simulink model "Simple_Joystick_CGN"  (R2025b)
settings: Solver=FixedStepDiscrete  StartTime=0.0  StopTime=inf  RelTol=1e-3
undefined symbols (not defined in the file): pwm_zero_set
libraries: ros2lib x2
settings Model: Creator=vulcangrip  LastModifiedBy=vulcangrip
settings OptimizationCC: DefaultParameterBehavior=Inlined  EnhancedBackFolding=on  PassReuseOutputArgsAs=Individual arguments  ZeroExternalMemoryAtStartup=off  ZeroInternalMemoryAtStartup=off  MaxStackSize=64  OptimizeBlockOrder=speed  DifferentSizesBufferReuse=on  OptimizationCustomize=off  EfficientTunableParamExpr=on
settings DebuggingCC: ParameterTunabilityLossMsg=error
settings HardwareCC: ProdBitPerLong=64.0  ProdHWDeviceType=Intel->x86-64 (Linux 64)
settings SFSimCC: MATLABDynamicMemAlloc=off  SimTargetLang=C++  SimDLTargetLibrary=mkl-dnn
settings RTWCC: SystemTargetFile=ert.tlc  HardwareBoard=Robot Operating System 2 (ROS 2)  TLCOptions="-aInlineSetEventsForThisBaseRateFcn=TLC_FALSE -aSuppressMultiTaskScheduler=TLC_FALSE  -aRateBasedStepFcn=0"  GenCodeOnly=on  TemplateMakefile=ert_default_tmf  Toolchain=Colcon Tools  BuildConfiguration=Faster Runs  TargetLang=C++  CheckMdlBeforeBuild=Warning  Description=Embedded Coder
settings CodeAppCC: ForceParamTrailComments=on  IgnoreCustomStorageClasses=off  OperatorAnnotations=on  SimulinkDataObjDesc=on  SFDataObjDesc=on  InsertBlockDesc=on
settings ERTTargetCC: ExtModeTransport=2.0  ExtModeStaticAlloc=on  ExtModeAutomaticAllocSize=off  ExtModeMexFile=ext_xcp  ExtModeIntrfLevel=Level2 - Open  RootIOFormat=Structure reference  TargetLangStandard=C++11 (ISO)  CodeInterfacePackaging=C++ class  SubcomponentCodeInterfacePackaging=C++ class

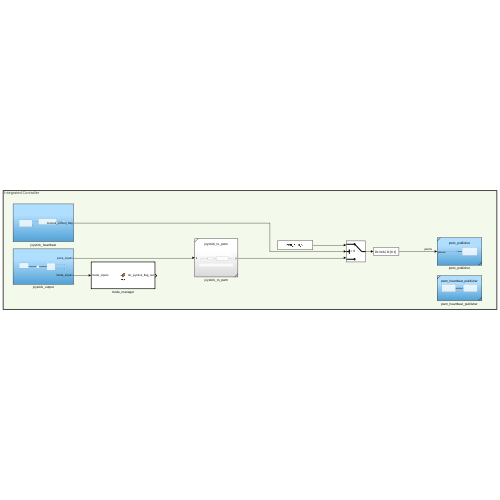
[thumbnail: Simulink's stored preview of the top-level diagram]
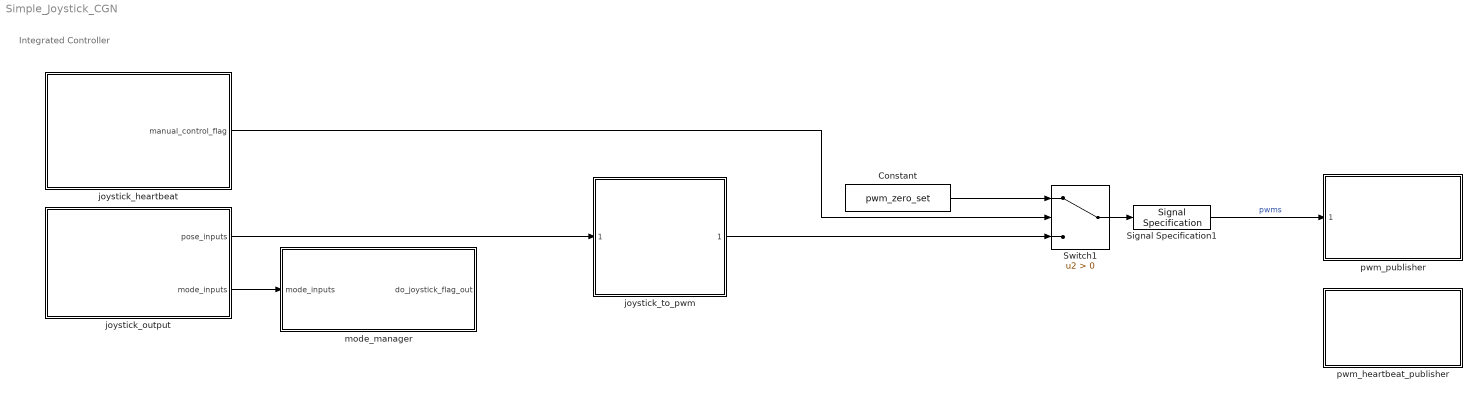
== system Simple_Joystick_CGN ==
  note: Integrated Controller
  Constant : Constant  Value=pwm_zero_set  OutDataTypeStr=int32
  Signal Specification1 : SignalSpecification  OutDataTypeStr=int32  Dimensions=[8 1]
  Switch1 : Switch  Criteria=u2 > Threshold  SaturateOnIntegerOverflow=off  InputSameDT=off
  joystick_heartbeat : Subsystem
  joystick_output : Subsystem
  joystick_to_pwm : Subsystem  ReferencedSubsystem=joystick_to_pwm
  mode_manager : MATLAB Function  TreatAsAtomicUnit=on
  pwm_heartbeat_publisher : Subsystem  ReferencedSubsystem=pwm_heartbeat_publisher
  pwm_publisher : Subsystem  ReferencedSubsystem=pwm_publisher
  wires:
  Constant/1 -> Switch1/1
  joystick_heartbeat/1(manual_control_flag) -> Switch1/2
  joystick_to_pwm/1 -> Switch1/3
  Switch1/1 -> Signal Specification1/1
  joystick_output/2(mode_inputs) -> mode_manager/1(mode_inputs)
  joystick_output/1(pose_inputs) -> joystick_to_pwm/1
  Signal Specification1/1 -> pwm_publisher/1  "pwms"

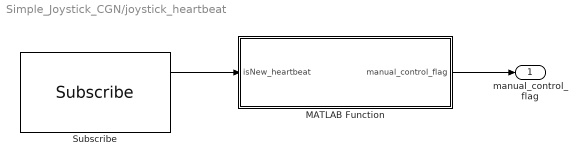
== system Simple_Joystick_CGN/joystick_heartbeat ==
  MATLAB Function : MATLAB Function  TreatAsAtomicUnit=on
  Subscribe : ros2lib/Subscribe  topicSource=Select from ROS network  topic=/joystick_heartbeat  messageType=std_msgs/Empty  sampleTime=-1  QOSHistory=Keep last  QOSDepth=10  QOSReliability=Reliable  QOSDurability=Volatile  QOSDeadline=Inf  QOSLifespan=Inf  QOSLiveliness=Automatic  QOSLeaseDuration=Inf  QOSAvoidROSNamespaceConventions=off
  manual_control_flag : Outport
  wires:
  Subscribe/1 -> MATLAB Function/1(isNew_heartbeat)
  MATLAB Function/1(manual_control_flag) -> manual_control_flag/1

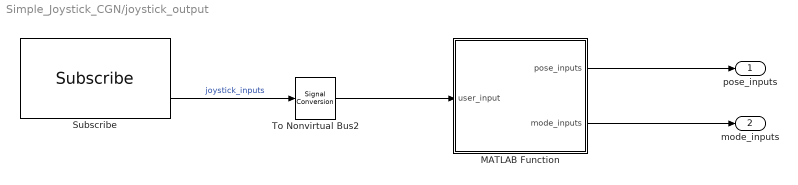
== system Simple_Joystick_CGN/joystick_output ==
  MATLAB Function : MATLAB Function  TreatAsAtomicUnit=on
  Subscribe : ros2lib/Subscribe  topicSource=Specify your own  topic=/ps5_controller  messageType=custom_interfaces/Gamepad  sampleTime=1/100  QOSHistory=Keep last  QOSDepth=10  QOSReliability=Reliable  QOSDurability=Volatile  QOSDeadline=Inf  QOSLifespan=Inf  QOSLiveliness=Automatic  QOSLeaseDuration=Inf  QOSAvoidROSNamespaceConventions=off
  To Nonvirtual Bus2 : SignalConversion  ConversionOutput=Nonvirtual bus  OutDataTypeStr=Bus: SL_Bus_custom_interfaces_Gamepad  OverrideOpt=off
  pose_inputs : Outport
  mode_inputs : Outport  Port=2
  wires:
  Subscribe/2 -> To Nonvirtual Bus2/1  "joystick_inputs"
  To Nonvirtual Bus2/1 -> MATLAB Function/1(user_input)
  MATLAB Function/1(pose_inputs) -> pose_inputs/1
  MATLAB Function/2(mode_inputs) -> mode_inputs/1

== matlab function Simple_Joystick_CGN/joystick_heartbeat/MATLAB Function ==
  data: isNew_heartbeat input boolean; manual_control_flag output boolean; dt_control parameter
function manual_control_flag = fcn(isNew_heartbeat,dt_control)

manual_control_flag = heartbeat_interpreter(isNew_heartbeat,dt_control);

== matlab function Simple_Joystick_CGN/joystick_output/MATLAB Function ==
  data: user_input input; pose_inputs output; mode_inputs output
function [pose_inputs, mode_inputs] = fcn(user_input)

[pose_inputs, mode_inputs] = gamepad_parser(user_input);

== matlab function Simple_Joystick_CGN/mode_manager ==
  data: mode_inputs input; do_joystick_flag_out output
function do_joystick_flag_out   = fcn(mode_inputs)
    
[do_joystick_flag_out,~] = mode_manager(mode_inputs);
